simulink model "SIR2"  (R2020a)
settings: Solver=VariableStepAuto  StartTime=0.0  StopTime=300  RelTol=1e-3
values from neighbouring files (symbols this model uses):
  be = 1.860000000000000    (= 1.86)    [COVID19.m]
  c = 1-0.984    (= 0.016)    [COVID19.m]
  ga = 1.780000000000000    (= 1.78)    [COVID19.m]
  i0 = 1/N    (= 2.77777777778e-08)    [COVID19.m]
  r0 = 0    [COVID19.m]
  s0 = 1-i0-r0    (= 0.999999972222)    [COVID19.m]
settings Model: Creator=Houda Assad

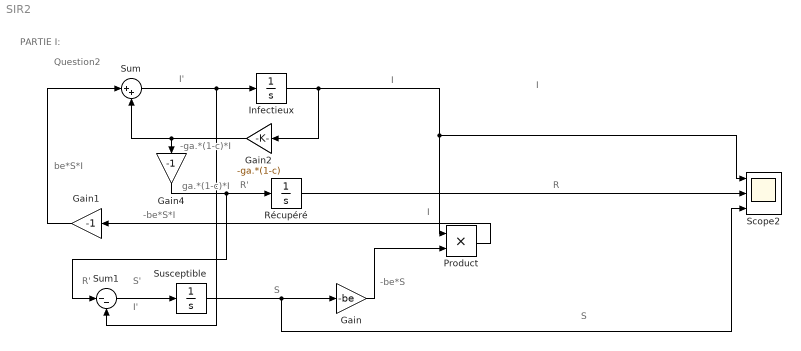
== system SIR2 ==
  note: Question2
  note: I'
  note: R'
  note: ga.*(1-c)*I
  note: be*S*I
  note: -be*S*I
  note: I
  note: S
  note: I
  note: I'
  note: R'
  note: S'
  note: -be*S
  note: R
  note: -ga.*(1-c)*I
  note: I
  note: S
  note: PARTIE I:
  Gain : Gain  Gain=-be
  Gain1 : Gain  Gain=-1
  Gain2 : Gain  Gain=-ga.*(1-c)
  Gain4 : Gain  Gain=-1
  Infectieux : Integrator  InitialCondition=i0
  Product : Product
  Récupéré : Integrator  InitialCondition=r0
  Scope2 : Scope  NumInputPorts=3
  Sum : Sum  Inputs=|++
  Sum1 : Sum  Inputs=|--
  Susceptible : Integrator  InitialCondition=s0
  wires:
  Susceptible/1 -> Scope2/3, Gain/1
  Gain2/1 -> Gain4/1, Sum/2
  Gain1/1 -> Sum/1
  Gain/1 -> Product/2
  Product/1 -> Gain1/1
  Infectieux/1 -> Gain2/1, Scope2/1, Product/1
  Récupéré/1 -> Scope2/2
  Gain4/1 -> Sum1/1, Récupéré/1
  Sum1/1 -> Susceptible/1
  Sum/1 -> Sum1/2, Infectieux/1
